simulink library "ctrl_L1_angular_rate"  (R2019b)
settings: Solver=VariableStepAuto  StartTime=0.0  StopTime=10.0  RelTol=1e-3
libraries: simulink x4, cal_eata x1
settings Model: Creator=Huitao Lv  LastModifiedBy=75696
settings DataIOCC: ReturnWorkspaceOutputs=off
settings DebuggingCC: ArithmeticOperatorsInVariantConditions=warning
settings SFSimCC: CustomCodeUndefinedFunction=UseInterfaceOnly

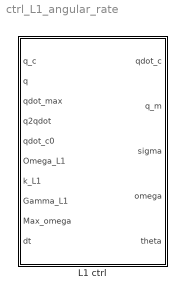
== system ctrl_L1_angular_rate ==
  L1 ctrl : Subsystem  mask(L1 adapative control){}
      mask help:
      | L1 adaptive control algorithm
      | for innerloop angular rate control
      mask Display:
      | port_label('input',1,'q_c', 'texmode', 'on');
      | port_label('input',2,'q', 'texmode', 'off');
      | port_label('input',3,'qdot_{max}', 'texmode', 'on');
      | port_label('input',4,'qdot_q', 'texmode', 'on');
      | port_label('input',5,'qdot_{c0}', 'texmode', 'on');
      | port_label('input',6,'Omega_{L1}', 'texmode', 'on');
      | port_label('input',7,'k_{L1}', 'texmode', 'on');
      | port_label('input',8,'Gamma_{L1}', 'texmode', 'on');
      | port_label('input',9,'Max_{omega}', 'texmode', 'on');
      | port_label('input',10,'dt', 'texmode', 'on');
      | port_label('output',1,'qdot_c', 'texmode', 'on');
      | port_label('output',2,'q_{hat}', 'texmode', 'on');
      | port_label('output',3,'\sigma_{hat}', 'texmode', 'on');
      | port_label('output',4,'\omega_{hat}', 'texmode', 'on');
      | port_label('output',5,'\theta_{hat}', 'texmode', 'on');
      | disp('L1 adaptor ctrl');

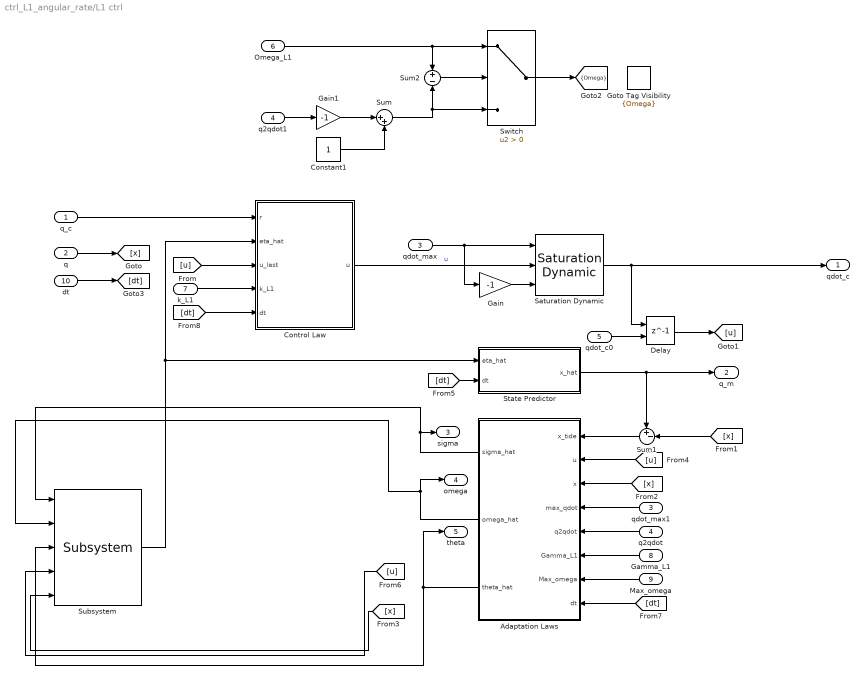
== system ctrl_L1_angular_rate/L1 ctrl ==
  q_c : Inport
  q : Inport  Port=2
  qdot_max : Inport  Port=3
  q2qdot : Inport  Port=4
  qdot_c0 : Inport  Port=5
  Omega_L1 : Inport  Port=6
  k_L1 : Inport  Port=7
  Gamma_L1 : Inport  Port=8
  Max_omega : Inport  Port=9
  dt : Inport  Port=10
  Adaptation Laws : Subsystem
  Constant1 : Constant  OutDataTypeStr=single
  Control Law : Subsystem
  Delay : Delay  DelayLength=1  InitialConditionSource=Input port
      settings: InputPortMap=u0,p4
  Gain : Gain  Gain=-1
  Gain1 : Gain  Gain=-1
  Goto Tag Visibility : GotoTagVisibility  GotoTag=Omega
  Saturation Dynamic : simulink/Discontinuities/Saturation Dynamic  OutMin=[]  OutMax=[]  OutDataTypeStr=single  OutputDataTypeScalingMode=single  OutDataType=fixdt(1, 16)  OutScaling=2^-10  DoSatur=off
  State Predictor : Subsystem
  Subsystem : cal_eata/Subsystem  SystemSampleTime=-1  Latency=0  AutoFrameSizeCalculation=off
  Sum : Sum  Inputs=|++
  Sum1 : Sum  Inputs=+-|
  Sum2 : Sum  Inputs=+|-
  Switch : Switch  Criteria=u2 > Threshold
  q2qdot1 : InportShadow  Port=4
  qdot_max1 : InportShadow  Port=3
  qdot_c : Outport  VectorParamsAs1DForOutWhenUnconnected=off
  q_m : Outport  Port=2  VectorParamsAs1DForOutWhenUnconnected=off
  sigma : Outport  Port=3  VectorParamsAs1DForOutWhenUnconnected=off
  omega : Outport  Port=4  VectorParamsAs1DForOutWhenUnconnected=off
  theta : Outport  Port=5  VectorParamsAs1DForOutWhenUnconnected=off
  tag scope: Omega=scoped
  wires:
  Gain/1 -> Saturation Dynamic/3
  Adaptation Laws/1(sigma_hat) -> Subsystem/1, sigma/1
  q2qdot1/1 -> Gain1/1
  Constant1/1 -> Sum/2
  [u] -> Subsystem/4
  State Predictor/1(x_hat) -> q_m/1, Sum1/1
  Sum1/1 -> Adaptation Laws/1(x_tide)
  [x] -> Sum1/2
  Delay/1 -> [u]
  [x] -> Adaptation Laws/3(x)
  q/1 -> [x]
  Adaptation Laws/3(theta_hat) -> theta/1, Subsystem/3
  Subsystem/1 -> Control Law/2(eta_hat), State Predictor/1(eta_hat)
  [u] -> Adaptation Laws/2(u)
  q_c/1 -> Control Law/1(r)
  [u] -> Control Law/3(u_last)
  Control Law/1(u) -> Saturation Dynamic/2  "u"
  Omega_L1/1 -> Switch/1, Sum2/1
  [x] -> Subsystem/5
  Sum/1 -> Sum2/2, Switch/3
  q2qdot/1 -> Adaptation Laws/5(q2qdot)
  qdot_max1/1 -> Adaptation Laws/4(max_qdot)
  Saturation Dynamic/1 -> qdot_c/1, Delay/1
  qdot_max/1 -> Gain/1, Saturation Dynamic/1
  Sum2/1 -> Switch/2
  Switch/1 -> [Omega]
  Gain1/1 -> Sum/1
  qdot_c0/1 -> Delay/2
  Adaptation Laws/2(omega_hat) -> Subsystem/2, omega/1
  dt/1 -> [dt]
  [dt] -> State Predictor/2(dt)
  [dt] -> Adaptation Laws/8(dt)
  [dt] -> Control Law/5(dt)
  k_L1/1 -> Control Law/4(k_L1)
  Gamma_L1/1 -> Adaptation Laws/6(Gamma_L1)
  Max_omega/1 -> Adaptation Laws/7(Max_omega)

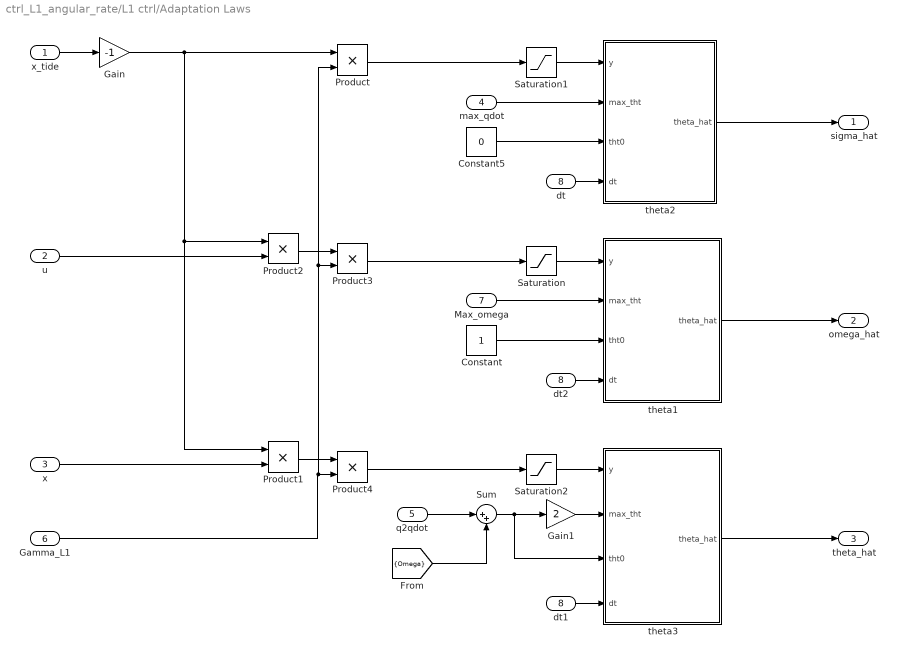
== system ctrl_L1_angular_rate/L1 ctrl/Adaptation Laws ==
  x_tide : Inport
  u : Inport  Port=2
  x : Inport  Port=3
  max_qdot : Inport  Port=4
  q2qdot : Inport  Port=5
  Gamma_L1 : Inport  Port=6
  Max_omega : Inport  Port=7
  dt : Inport  Port=8
  Constant : Constant  OutDataTypeStr=single
  Constant5 : Constant  Value=0  OutDataTypeStr=single
  Gain : Gain  Gain=-1
  Gain1 : Gain  Gain=2
  Product{,1..4} (5 alike) : Product
  Saturation : Saturate  UpperLimit=1000  LowerLimit=-1000
  Saturation1 : Saturate  UpperLimit=1000  LowerLimit=-1000
  Saturation2 : Saturate  UpperLimit=1000  LowerLimit=-1000
  Sum : Sum  Inputs=|++
  dt1 : InportShadow  Port=8
  dt2 : InportShadow  Port=8
  theta1 : Subsystem  TreatAsAtomicUnit=on
  theta2 : Subsystem  TreatAsAtomicUnit=on
  theta3 : Subsystem  TreatAsAtomicUnit=on
  sigma_hat : Outport  VectorParamsAs1DForOutWhenUnconnected=off
  omega_hat : Outport  Port=2  VectorParamsAs1DForOutWhenUnconnected=off
  theta_hat : Outport  Port=3  VectorParamsAs1DForOutWhenUnconnected=off
  wires:
  Product/1 -> Saturation1/1
  Product3/1 -> Saturation/1
  Product2/1 -> Product3/1
  u/1 -> Product2/2
  x_tide/1 -> Gain/1
  Gain/1 -> Product/1, Product1/1, Product2/1
  x/1 -> Product1/2
  Product1/1 -> Product4/1
  Product4/1 -> Saturation2/1
  theta3/1(theta_hat) -> theta_hat/1
  theta1/1(theta_hat) -> omega_hat/1
  theta2/1(theta_hat) -> sigma_hat/1
  Constant/1 -> theta1/3(tht0)
  Sum/1 -> Gain1/1, theta3/3(tht0)
  Max_omega/1 -> theta1/2(max_tht)
  Constant5/1 -> theta2/3(tht0)
  max_qdot/1 -> theta2/2(max_tht)
  Gain1/1 -> theta3/2(max_tht)
  q2qdot/1 -> Sum/1
  [Omega] -> Sum/2
  Saturation/1 -> theta1/1(y)
  Saturation1/1 -> theta2/1(y)
  Saturation2/1 -> theta3/1(y)
  Gamma_L1/1 -> Product/2, Product3/2, Product4/2
  dt/1 -> theta2/4(dt)
  dt1/1 -> theta3/4(dt)
  dt2/1 -> theta1/4(dt)

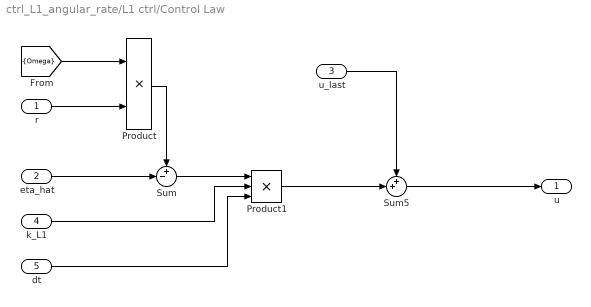
== system ctrl_L1_angular_rate/L1 ctrl/Control Law ==
  r : Inport
  eta_hat : Inport  Port=2
  u_last : Inport  Port=3
  k_L1 : Inport  Port=4
  dt : Inport  Port=5
  Product : Product
  Product1 : Product  Inputs=3
  Sum : Sum  Inputs=+-|
  Sum5 : Sum  Inputs=++|
  u : Outport  VectorParamsAs1DForOutWhenUnconnected=off
  wires:
  eta_hat/1 -> Sum/2
  Sum/1 -> Product1/1
  Sum5/1 -> u/1
  Product1/1 -> Sum5/2
  r/1 -> Product/2
  Product/1 -> Sum/1
  [Omega] -> Product/1
  u_last/1 -> Sum5/1
  k_L1/1 -> Product1/2
  dt/1 -> Product1/3

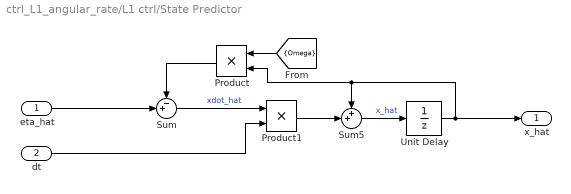
== system ctrl_L1_angular_rate/L1 ctrl/State Predictor ==
  eta_hat : Inport
  dt : Inport  Port=2
  Product : Product
  Product1 : Product
  Sum : Sum  Inputs=-+|
  Sum5 : Sum  Inputs=++|
  Unit Delay : UnitDelay  SampleTime=-1  HasFrameUpgradeWarning=on
  x_hat : Outport  VectorParamsAs1DForOutWhenUnconnected=off
  wires:
  Product1/1 -> Sum5/2
  Sum5/1 -> Unit Delay/1  "x_hat"
  Sum/1 -> Product1/1  "xdot_hat"
  Product/1 -> Sum/1
  eta_hat/1 -> Sum/2
  Unit Delay/1 -> Sum5/1, Product/2, x_hat/1
  [Omega] -> Product/1
  dt/1 -> Product1/2

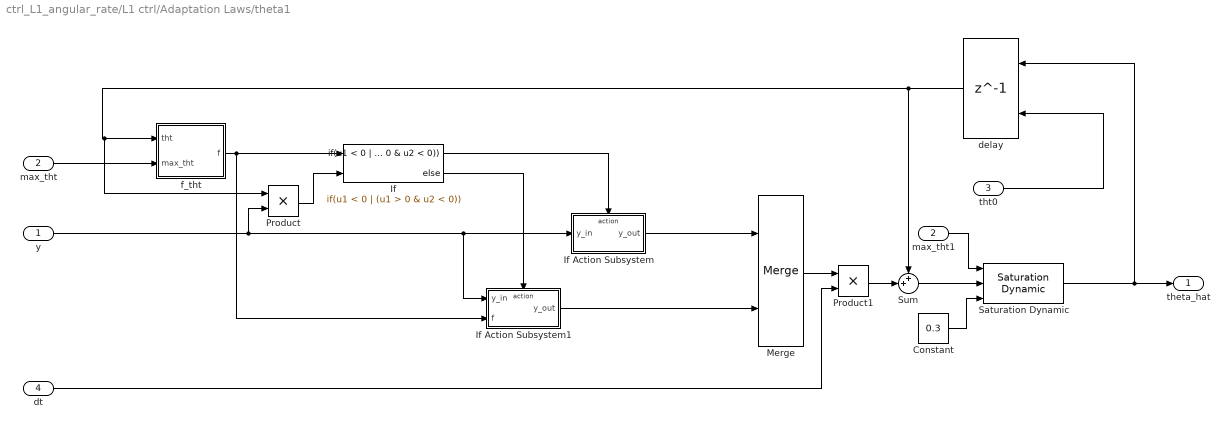
== system ctrl_L1_angular_rate/L1 ctrl/Adaptation Laws/theta1 ==
  y : Inport
  max_tht : Inport  Port=2
  tht0 : Inport  Port=3
  dt : Inport  Port=4
  Constant : Constant  Value=0.3  OutDataTypeStr=Inherit: Inherit via back propagation
  If : If  NumInputs=2  IfExpression=u1 < 0 | (u1 > 0 & u2 < 0)
  If Action Subsystem : Subsystem  TreatAsAtomicUnit=on
  If Action Subsystem1 : Subsystem  TreatAsAtomicUnit=on
  Merge : Merge
  Product : Product
  Product1 : Product
  Saturation Dynamic : simulink/Discontinuities/Saturation Dynamic  OutMin=[]  OutMax=[]  OutDataTypeStr=Inherit: Same as second input  OutDataType=fixdt(1, 16)  OutScaling=2^-10  DoSatur=off
  Sum : Sum  Inputs=++|
  delay : Delay  DelayLength=1  InitialConditionSource=Input port
      settings: InputPortMap=u0,p4
  f_tht : Subsystem
  max_tht1 : InportShadow  Port=2
  theta_hat : Outport  VectorParamsAs1DForOutWhenUnconnected=off
  wires:
  tht0/1 -> delay/2
  Saturation Dynamic/1 -> delay/1, theta_hat/1
  Product1/1 -> Sum/2
  Merge/1 -> Product1/1
  max_tht/1 -> f_tht/2(max_tht)
  If/2 -> If Action Subsystem1/Action
  If Action Subsystem1/1(y_out) -> Merge/2
  delay/1 -> f_tht/1(tht), Product/1, Sum/1
  y/1 -> If Action Subsystem/1(y_in), If Action Subsystem1/1(y_in), Product/2
  If Action Subsystem/1(y_out) -> Merge/1
  If/1 -> If Action Subsystem/Action
  Product/1 -> If/2
  f_tht/1(f) -> If/1, If Action Subsystem1/2(f)
  Sum/1 -> Saturation Dynamic/2
  max_tht1/1 -> Saturation Dynamic/1
  Constant/1 -> Saturation Dynamic/3
  dt/1 -> Product1/2

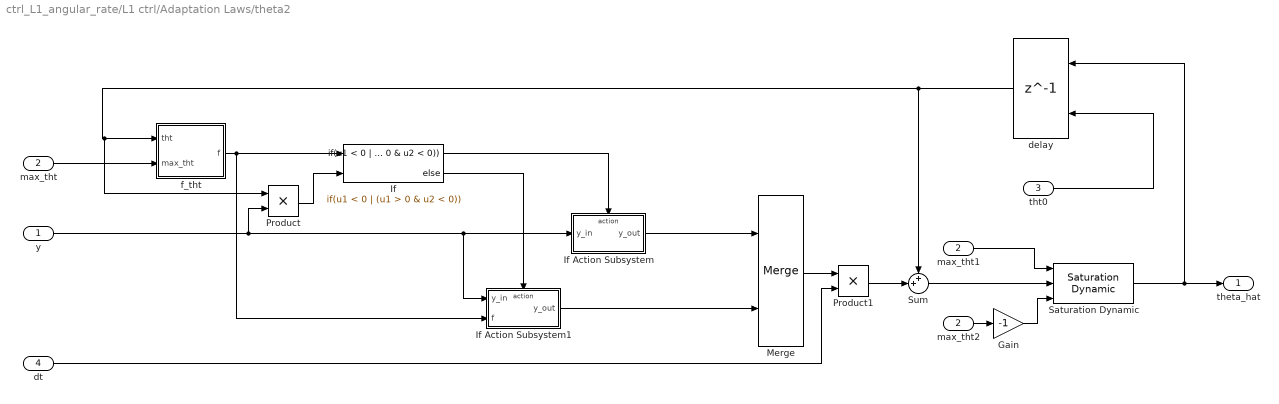
== system ctrl_L1_angular_rate/L1 ctrl/Adaptation Laws/theta2 ==
  y : Inport
  max_tht : Inport  Port=2
  tht0 : Inport  Port=3
  dt : Inport  Port=4
  Gain : Gain  Gain=-1
  If : If  NumInputs=2  IfExpression=u1 < 0 | (u1 > 0 & u2 < 0)
  If Action Subsystem : Subsystem  TreatAsAtomicUnit=on
  If Action Subsystem1 : Subsystem  TreatAsAtomicUnit=on
  Merge : Merge
  Product : Product
  Product1 : Product
  Saturation Dynamic : simulink/Discontinuities/Saturation Dynamic  OutMin=[]  OutMax=[]  OutDataTypeStr=Inherit: Same as second input  OutDataType=fixdt(1, 16)  OutScaling=2^-10  DoSatur=off
  Sum : Sum  Inputs=++|
  delay : Delay  DelayLength=1  InitialConditionSource=Input port
      settings: InputPortMap=u0,p4
  f_tht : Subsystem
  max_tht1 : InportShadow  Port=2
  max_tht2 : InportShadow  Port=2
  theta_hat : Outport  VectorParamsAs1DForOutWhenUnconnected=off
  wires:
  f_tht/1(f) -> If Action Subsystem1/2(f), If/1
  Product/1 -> If/2
  If/1 -> If Action Subsystem/Action
  If Action Subsystem/1(y_out) -> Merge/1
  y/1 -> Product/2, If Action Subsystem1/1(y_in), If Action Subsystem/1(y_in)
  delay/1 -> Sum/1, Product/1, f_tht/1(tht)
  If Action Subsystem1/1(y_out) -> Merge/2
  If/2 -> If Action Subsystem1/Action
  max_tht/1 -> f_tht/2(max_tht)
  Merge/1 -> Product1/1
  Product1/1 -> Sum/2
  Saturation Dynamic/1 -> theta_hat/1, delay/1
  tht0/1 -> delay/2
  Sum/1 -> Saturation Dynamic/2
  max_tht1/1 -> Saturation Dynamic/1
  max_tht2/1 -> Gain/1
  Gain/1 -> Saturation Dynamic/3
  dt/1 -> Product1/2

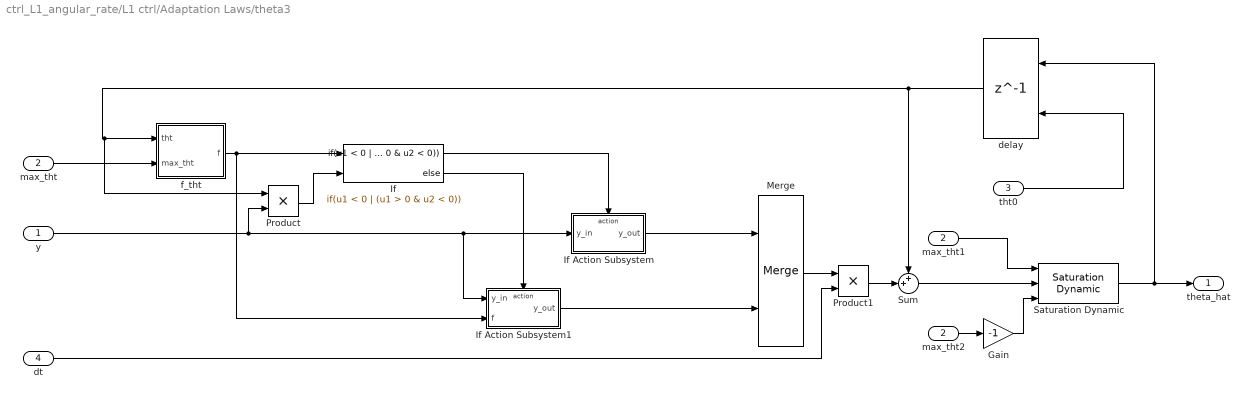
== system ctrl_L1_angular_rate/L1 ctrl/Adaptation Laws/theta3 ==
  y : Inport
  max_tht : Inport  Port=2
  tht0 : Inport  Port=3
  dt : Inport  Port=4
  Gain : Gain  Gain=-1
  If : If  NumInputs=2  IfExpression=u1 < 0 | (u1 > 0 & u2 < 0)
  If Action Subsystem : Subsystem  TreatAsAtomicUnit=on
  If Action Subsystem1 : Subsystem  TreatAsAtomicUnit=on
  Merge : Merge
  Product : Product
  Product1 : Product
  Saturation Dynamic : simulink/Discontinuities/Saturation Dynamic  OutMin=[]  OutMax=[]  OutDataTypeStr=Inherit: Same as second input  OutDataType=fixdt(1, 16)  OutScaling=2^-10  DoSatur=off
  Sum : Sum  Inputs=++|
  delay : Delay  DelayLength=1  InitialConditionSource=Input port
      settings: InputPortMap=u0,p4
  f_tht : Subsystem
  max_tht1 : InportShadow  Port=2
  max_tht2 : InportShadow  Port=2
  theta_hat : Outport  VectorParamsAs1DForOutWhenUnconnected=off
  wires:
  Gain/1 -> Saturation Dynamic/3
  max_tht2/1 -> Gain/1
  max_tht1/1 -> Saturation Dynamic/1
  Sum/1 -> Saturation Dynamic/2
  tht0/1 -> delay/2
  Saturation Dynamic/1 -> delay/1, theta_hat/1
  Product1/1 -> Sum/2
  Merge/1 -> Product1/1
  max_tht/1 -> f_tht/2(max_tht)
  If/2 -> If Action Subsystem1/Action
  If Action Subsystem1/1(y_out) -> Merge/2
  delay/1 -> f_tht/1(tht), Product/1, Sum/1
  y/1 -> If Action Subsystem/1(y_in), If Action Subsystem1/1(y_in), Product/2
  If Action Subsystem/1(y_out) -> Merge/1
  If/1 -> If Action Subsystem/Action
  Product/1 -> If/2
  f_tht/1(f) -> If/1, If Action Subsystem1/2(f)
  dt/1 -> Product1/2

== system ctrl_L1_angular_rate/L1 ctrl/Adaptation Laws/theta1/If Action Subsystem ==
  y_in : Inport
  Action Port : ActionPort
  y_out : Outport  VectorParamsAs1DForOutWhenUnconnected=off
  wires:
  y_in/1 -> y_out/1

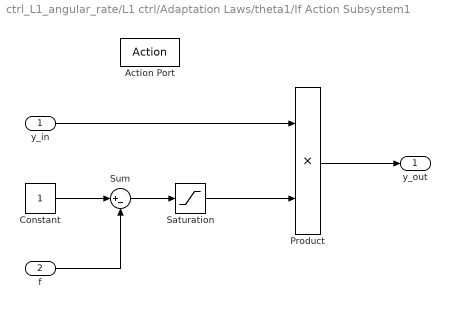
== system ctrl_L1_angular_rate/L1 ctrl/Adaptation Laws/theta1/If Action Subsystem1 ==
  y_in : Inport
  f : Inport  Port=2
  Action Port : ActionPort
  Constant : Constant  OutDataTypeStr=single
  Product : Product
  Saturation : Saturate  UpperLimit=Inf  LowerLimit=0
  Sum : Sum  Inputs=|+-
  y_out : Outport  VectorParamsAs1DForOutWhenUnconnected=off
  wires:
  Saturation/1 -> Product/2
  Sum/1 -> Saturation/1
  f/1 -> Sum/2
  Constant/1 -> Sum/1
  y_in/1 -> Product/1
  Product/1 -> y_out/1

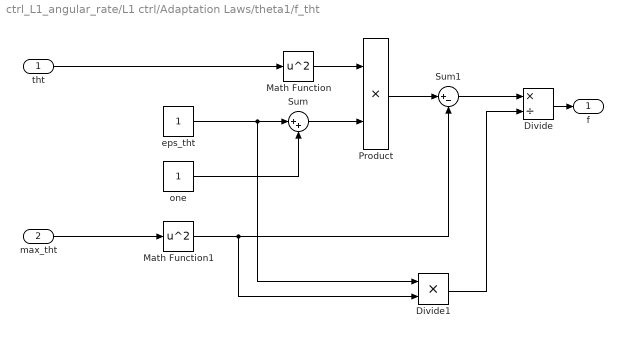
== system ctrl_L1_angular_rate/L1 ctrl/Adaptation Laws/theta1/f_tht ==
  tht : Inport
  max_tht : Inport  Port=2
  Divide : Product  Inputs=*/
  Divide1 : Product  Inputs=**
  Math Function : Math  Operator=square  SaturateOnIntegerOverflow=on
  Math Function1 : Math  Operator=square  SaturateOnIntegerOverflow=on
  Product : Product
  Sum : Sum  Inputs=|++
  Sum1 : Sum  Inputs=|+-
  eps_tht : Constant  OutDataTypeStr=single
  one : Constant  OutDataTypeStr=single
  f : Outport  VectorParamsAs1DForOutWhenUnconnected=off
  wires:
  Divide1/1 -> Divide/2
  Product/1 -> Sum1/1
  Math Function1/1 -> Sum1/2, Divide1/2
  Sum/1 -> Product/2
  eps_tht/1 -> Sum/1, Divide1/1
  Divide/1 -> f/1
  tht/1 -> Math Function/1
  Sum1/1 -> Divide/1
  max_tht/1 -> Math Function1/1
  Math Function/1 -> Product/1
  one/1 -> Sum/2

== system ctrl_L1_angular_rate/L1 ctrl/Adaptation Laws/theta2/If Action Subsystem ==
  y_in : Inport
  Action Port : ActionPort
  y_out : Outport  VectorParamsAs1DForOutWhenUnconnected=off
  wires:
  y_in/1 -> y_out/1

== system ctrl_L1_angular_rate/L1 ctrl/Adaptation Laws/theta2/If Action Subsystem1 ==
  y_in : Inport
  f : Inport  Port=2
  Action Port : ActionPort
  Constant : Constant  OutDataTypeStr=single
  Product : Product
  Saturation : Saturate  UpperLimit=Inf  LowerLimit=0
  Sum : Sum  Inputs=|+-
  y_out : Outport  VectorParamsAs1DForOutWhenUnconnected=off
  wires:
  Product/1 -> y_out/1
  y_in/1 -> Product/1
  Constant/1 -> Sum/1
  f/1 -> Sum/2
  Sum/1 -> Saturation/1
  Saturation/1 -> Product/2

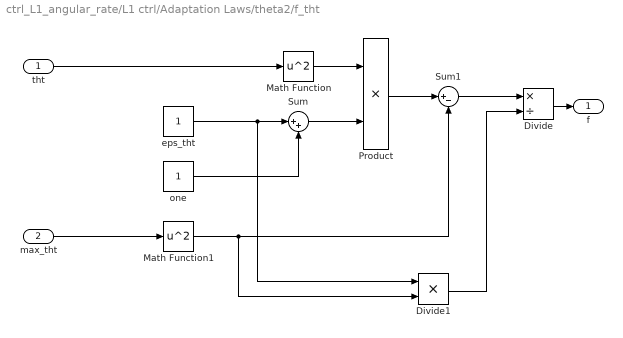
== system ctrl_L1_angular_rate/L1 ctrl/Adaptation Laws/theta2/f_tht ==
  tht : Inport
  max_tht : Inport  Port=2
  Divide : Product  Inputs=*/
  Divide1 : Product  Inputs=**
  Math Function : Math  Operator=square  SaturateOnIntegerOverflow=on
  Math Function1 : Math  Operator=square  SaturateOnIntegerOverflow=on
  Product : Product
  Sum : Sum  Inputs=|++
  Sum1 : Sum  Inputs=|+-
  eps_tht : Constant  OutDataTypeStr=single
  one : Constant  OutDataTypeStr=single
  f : Outport  VectorParamsAs1DForOutWhenUnconnected=off
  wires:
  one/1 -> Sum/2
  Math Function/1 -> Product/1
  max_tht/1 -> Math Function1/1
  Sum1/1 -> Divide/1
  tht/1 -> Math Function/1
  Divide/1 -> f/1
  eps_tht/1 -> Divide1/1, Sum/1
  Sum/1 -> Product/2
  Math Function1/1 -> Divide1/2, Sum1/2
  Product/1 -> Sum1/1
  Divide1/1 -> Divide/2

== system ctrl_L1_angular_rate/L1 ctrl/Adaptation Laws/theta3/If Action Subsystem ==
  y_in : Inport
  Action Port : ActionPort
  y_out : Outport  VectorParamsAs1DForOutWhenUnconnected=off
  wires:
  y_in/1 -> y_out/1

== system ctrl_L1_angular_rate/L1 ctrl/Adaptation Laws/theta3/If Action Subsystem1 ==
  y_in : Inport
  f : Inport  Port=2
  Action Port : ActionPort
  Constant : Constant  OutDataTypeStr=single
  Product : Product
  Saturation : Saturate  UpperLimit=Inf  LowerLimit=0
  Sum : Sum  Inputs=|+-
  y_out : Outport  VectorParamsAs1DForOutWhenUnconnected=off
  wires:
  Saturation/1 -> Product/2
  Sum/1 -> Saturation/1
  f/1 -> Sum/2
  Constant/1 -> Sum/1
  y_in/1 -> Product/1
  Product/1 -> y_out/1

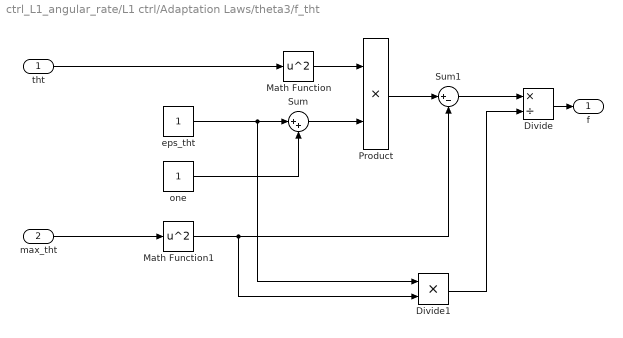
== system ctrl_L1_angular_rate/L1 ctrl/Adaptation Laws/theta3/f_tht ==
  tht : Inport
  max_tht : Inport  Port=2
  Divide : Product  Inputs=*/
  Divide1 : Product  Inputs=**
  Math Function : Math  Operator=square  SaturateOnIntegerOverflow=on
  Math Function1 : Math  Operator=square  SaturateOnIntegerOverflow=on
  Product : Product
  Sum : Sum  Inputs=|++
  Sum1 : Sum  Inputs=|+-
  eps_tht : Constant  OutDataTypeStr=single
  one : Constant  OutDataTypeStr=single
  f : Outport  VectorParamsAs1DForOutWhenUnconnected=off
  wires:
  Divide1/1 -> Divide/2
  Product/1 -> Sum1/1
  Math Function1/1 -> Sum1/2, Divide1/2
  Sum/1 -> Product/2
  eps_tht/1 -> Sum/1, Divide1/1
  Divide/1 -> f/1
  tht/1 -> Math Function/1
  Sum1/1 -> Divide/1
  max_tht/1 -> Math Function1/1
  Math Function/1 -> Product/1
  one/1 -> Sum/2
